simulink model "CD_simulink"  (R2024b)
settings: Solver=VariableStepAuto  StartTime=0.0  StopTime=0.01  RelTol=1e-3

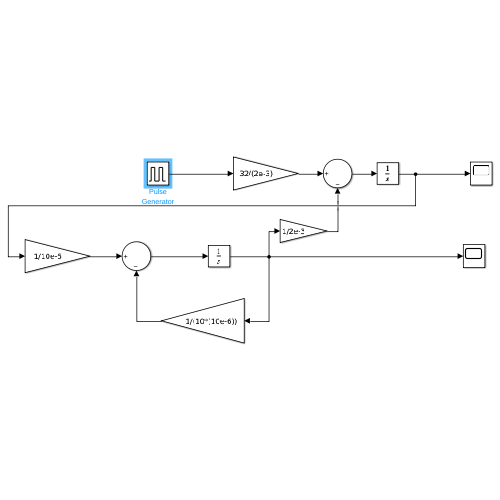
[thumbnail: Simulink's stored preview of the top-level diagram]
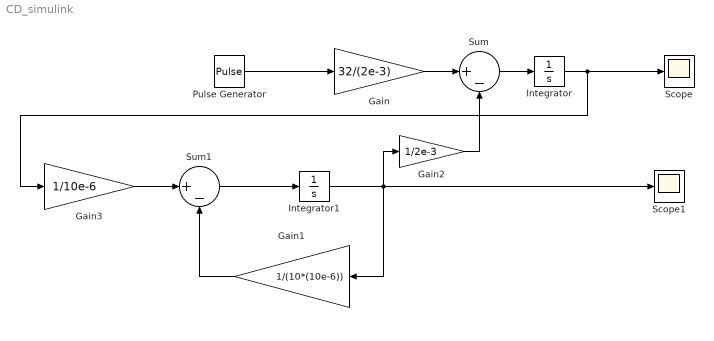
== system CD_simulink ==
  Gain : Gain  Gain=32/(2e-3)
  Gain1 : Gain  Gain=1/(10*(10e-6))
  Gain2 : Gain  Gain=1/2e-3
  Gain3 : Gain  Gain=1/10e-6
  Integrator : Integrator
  Integrator1 : Integrator
  Pulse Generator : DiscretePulseGenerator  PulseType=Time based  Period=1e-5  PulseWidth=50
  Scope : Scope
  Scope1 : Scope
  Sum : Sum  Inputs=|+-
  Sum1 : Sum  Inputs=|+-
  wires:
  Pulse Generator/1 -> Gain/1
  Gain/1 -> Sum/1
  Sum/1 -> Integrator/1
  Integrator/1 -> Gain3/1, Scope/1
  Gain2/1 -> Sum/2
  Gain1/1 -> Sum1/2
  Gain3/1 -> Sum1/1
  Sum1/1 -> Integrator1/1
  Integrator1/1 -> Gain1/1, Gain2/1, Scope1/1
